simulink model "firtest"  (Simulink 6.2)
settings: Solver=FixedStepDiscrete  SolverMode=SingleTasking  StartTime=0.0  StopTime=10240  RelTol=1e-3
libraries: xbsIndex_r3 x7, simulink x2, pfb_library x1
settings Model: LastModifiedBy=mdexter
settings DataIOCC: MaxDataPoints=20000
settings DebuggingCC: SolverPrmCheckMsg=warning

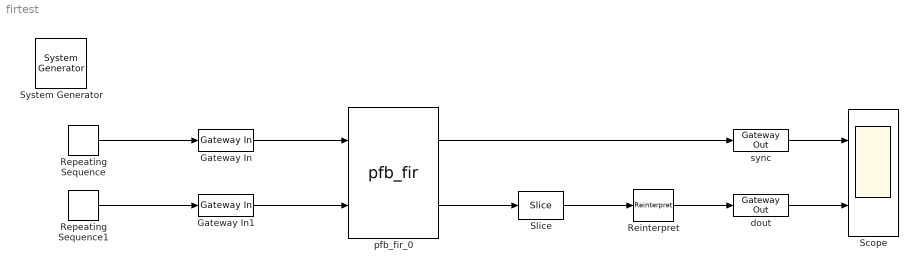
== system firtest ==
  " System Generator" : xbsIndex_r3/ System Generator  Tag=genX  xilinxfamily=Virtex2  part=xc2v1000  speed=-4  package=bg575  synthesis_tool=XST  directory=./netlist  testbench=off  simulink_period=1  sysclk_period=100  incr_netlist=off  trim_vbits=Everywhere in SubSystem  dbl_ovrd=According to Block Masks  core_generation=According to Block Masks  run_coregen=off  deprecated_control=off  eval_field=0
      settings: AttributesFormatString=System\nGenerator
  Gateway In : xbsIndex_r3/Gateway In  arith_type=Boolean  n_bits=8  bin_pt=6  quantization=Truncate  overflow=Wrap  period=1  timing_constraint=None  locs_specified=off  LOCs={}  needs_fixed_name=off  dbl_ovrd=off  show_param=off
      settings: xl_area=[0, 0, 0, 0, 0, 0, 0]
  Gateway In1 : xbsIndex_r3/Gateway In  arith_type=Unsigned  n_bits=16  bin_pt=0  quantization=Truncate  overflow=Wrap  period=1  timing_constraint=None  locs_specified=off  LOCs={}  needs_fixed_name=off  dbl_ovrd=off  show_param=off
      settings: xl_area=[0, 0, 0, 0, 0, 0, 0]
  Reinterpret : xbsIndex_r3/Reinterpret  force_arith_type=on  arith_type="Signed  (2's comp)"  force_bin_pt=on  bin_pt=0  force_valid=on
  Repeating Sequence : simulink/Sources/Repeating Sequence  rep_seq_t=[0:8192]  rep_seq_y=[1 zeros(1,8191) 1]
  Repeating Sequence1 : simulink/Sources/Repeating Sequence  rep_seq_t=[0:8192]  rep_seq_y=1*[0 ones(1,1024) zeros(1,7*1024)]
  Scope : Scope  NumInputPorts=2
      settings: YMin=0~0  YMax=1~7.5e+010  MaxDataPoints=20000
  Slice : xbsIndex_r3/Slice  mode=Lower Bit Location + Width  nbits=18  bit1=0  base1=LSB of Input  bit0=0  base0=LSB of Input  boolean_output=off  explicit_period=off  period=1  dbl_ovrd=off
  dout : xbsIndex_r3/Gateway Out  output_type=Double  nbits=8  bin_pt=6  arith_type=Boolean  quantization=Truncate  overflow=Wrap  hdl_port=on  timing_constraint=None  locs_specified=off  LOCs={}  needs_fixed_name=off  show_param=off
      settings: xl_area=[0, 0, 0, 0, 0, 0, 0]
  pfb_fir_0 : pfb_library/pfb_fir  PFBSize=10  TotalTaps=8  WindowType=hamming  n_inputs=0  MakeBiplex=off  BitWidthIn=8  BitWidthOut=18  CoeffBitWidth=8  CoeffDistMem=off  add_latency=2  mult_latency=3  bram_latency=2  quantization="Round  (unbiased: +/- Inf)"  fwidth=1
  sync : xbsIndex_r3/Gateway Out  output_type=Double  nbits=8  bin_pt=6  arith_type=Boolean  quantization=Truncate  overflow=Wrap  hdl_port=on  timing_constraint=None  locs_specified=off  LOCs={}  needs_fixed_name=off  show_param=off
      settings: xl_area=[0, 0, 0, 0, 0, 0, 0]
  wires:
  Gateway In/1 -> pfb_fir_0/1
  pfb_fir_0/1 -> sync/1
  pfb_fir_0/2 -> Slice/1
  Repeating Sequence/1 -> Gateway In/1
  Repeating Sequence1/1 -> Gateway In1/1
  sync/1 -> Scope/1
  dout/1 -> Scope/2
  Slice/1 -> Reinterpret/1
  Reinterpret/1 -> dout/1
  Gateway In1/1 -> pfb_fir_0/2
